simulink model "modelo_final_server"  (R2021a)
settings: Solver=FixedStepAuto  StartTime=0.0  StopTime=inf  FixedStep=0.001  MaxStep=1e-4  RelTol=1e-3
values from neighbouring files (symbols this model uses):
  bah = Meqh*nh*w_posh    (= 720000)    [Data.m]
  bat = Meqt*nt*w_post    (= 675000)    [Data.m]
  bcx = 1000.0    (= 1000)    [Data.m]
  bcy = 500.0    (= 500)    [Data.m]
  beqhd = bh + ((beqh*(rth^2))/(Rd^2))    (= 28800)    [Data.m]
  beqt = bt + (beq_rot*rt^2)/(Rw^2)    (= 27000)    [Data.m]
  bw = 30000.0    (= 30000)    [Data.m]
  cols_centers = [5,10,15,20,25,30,35,40,45]    [Data.m]    (also in generateTrajectory.m = ship.allocate_centers(container.width/2,delta))
  cols_height = [20,26,19,8,26,20,26,23,23]    [Data.m]    (also in generateTrajectory.m = ship.load(container))
  ddxmax = 1    [Data.m]
  ddxmin = -1    [Data.m]
  ddymax = 1    [Data.m]
  ddymin = -1    [Data.m]
  g = 9.80665    [Data.m]    (also in PD_balanceo.m = 9.81)
  Kcy = 1.3e6    (= 1300000)    [Data.m]
  Ksah = Meqh*nh*w_posh^2    (= 4318720.37915)    [Data.m]
  Ksat = Meqt*nt*w_post^2    (= 3088564.26247)    [Data.m]
  Ksiah = Meqh*w_posh^3    (= 10361858.7296)    [Data.m]
  Ksiat = Meqt*w_post^3    (= 5652876.56499)    [Data.m]
  Kw = 1800000.0    (= 1800000)    [Data.m]
  lh0 = yt0 - C_HEIGHT - 5 -(sp_mass * g) / Kw    (= 37.0282779167)    [Data.m]
  max_m = 50000.0    (= 50000)    [Data.m]
  Meqh = Mh + (Jmh*rth^2 + Jd)/Rd^2    (= 48014.2222222)    [Data.m]
  Meqt = mt + (Jw+Jm*rt^2)/(Rw^2)    (= 59008)    [Data.m]
  Rd = 0.75    [Data.m]
  rt = 15.0    (= 15)    [Data.m]    (also in main.m = 0)
  rth = 30.0    (= 30)    [Data.m]
  Rw = 0.5    [Data.m]    (also in main.m = 0)
  sp_mass = 15000.0    (= 15000)    [Data.m]
  w_mt_h = 1000    [Data.m]
  w_mt_i = 1000    [Data.m]
  xmax = 50    [Data.m]
  xt0 = -20    [Data.m]
  yt0 = 45.0    (= 45)    [Data.m]
undefined symbols (not defined in the file or in its folder): yl0
libraries: aerolibanimutils x1, simulink x1
settings Model: Creator=Mariano  LastModifiedBy=facu_
settings SolverCC: ODENIntegrationMethod=ode2

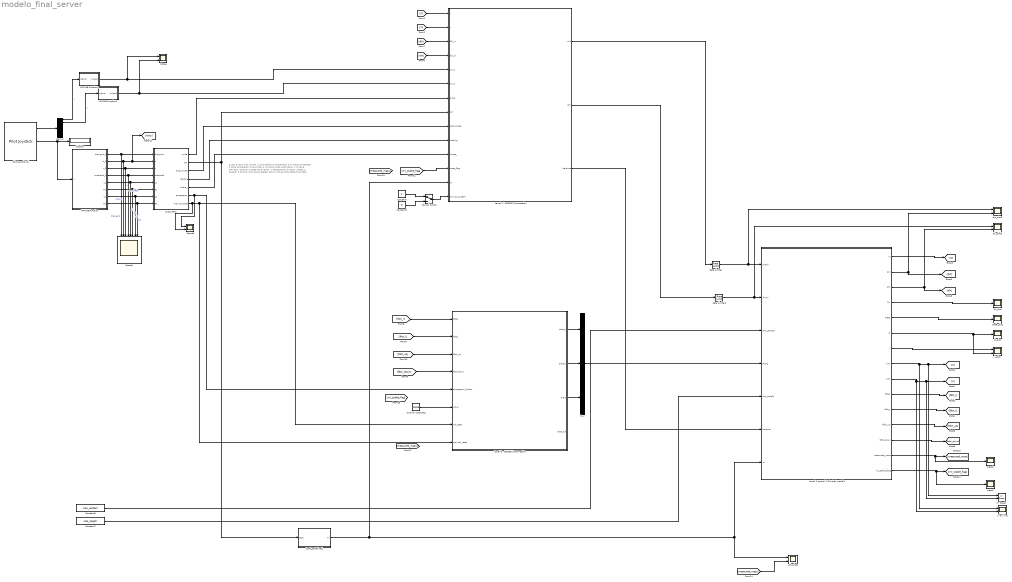
== system modelo_final_server ==
  note: Cycle: Si es 0 ciclo simple, 1 ciclo doble
      | twt (twtistlocks): 0 no tiene contenedor, 1 tiene contenedor.
      | auto_mode: 0 no tiene modo automatico, 1 lo tiene activado.
      | loading: 0 cargando el barco, 1 descargando el barco.
      | where_:1 to_dock, 0 to ship
      | manual_completed: tramo manual ciclo doble finalizado
  Constant : Constant
  Constant1 : Constant  Value=0
  Constant6 : Constant  Value=cols_centers
  Constant7 : Constant  Value=cols_height
  Demux : Demux  Outputs=6
  Display : Display
  Fw_plot : Scope
  Level 0 - CODESYS connection : Subsystem  TreatAsAtomicUnit=on  SystemSampleTime=0.1
  Level 1 - CODESYS connection : Subsystem  TreatAsAtomicUnit=on  SystemSampleTime=0.1
  Level 2 control + Physical model1 : Subsystem
  Load_container1 : Subsystem
  MATLAB Function : MATLAB Function  TreatAsAtomicUnit=on
  MATLAB Function1 : MATLAB Function  TreatAsAtomicUnit=on
  MATLAB Function2 : MATLAB Function  TreatAsAtomicUnit=on
  Manual Switch : ManualSwitch
  Mux : Mux  Inputs=3
  Pilot Joystick All : aerolibanimutils/Pilot Joystick  JoystickID=Joystick1  OutputConfiguration=AllOutputs  SampleTime=1/10
  Rate Limiter : RateLimiter  RisingSlewLimit=ddxmax  FallingSlewLimit=ddxmin  SampleTimeMode=inherited
  Rate Limiter1 : RateLimiter  RisingSlewLimit=ddymax  FallingSlewLimit=ddymin  SampleTimeMode=inherited
  Scope : Scope  NumInputPorts=2
  Scope1 : Scope  NumInputPorts=8
  Scope2 : Scope  NumInputPorts=2
  Subsystem : Subsystem
  XY Graph : simulink/Sinks/XY Graph  xmin=-22  xmax=50  ymin=0  ymax=50  st=-1
  clock for watchdog : DiscretePulseGenerator  PulseType=Time based  Period=1  PulseWidth=50
  dlh_plot1 : Scope  NumInputPorts=2
  dlh_plot2 : Scope  NumInputPorts=2
  dxt_plot3 : Scope  NumInputPorts=2
  l_plot : Scope  NumInputPorts=2
  lh_plot : Scope
  mass1 : Scope
  mass2 : Scope
  theta_plot : Scope
  xl e yl vs t : Scope  NumInputPorts=2
  wires:
  MATLAB Function/8(R2) -> Subsystem/8(R2), Scope1/8  "R2"
  MATLAB Function/7(L2) -> Subsystem/7(L2), Scope1/7  "L2"
  MATLAB Function/2(o_2) -> Scope1/2, [twts], Subsystem/2(o)  "circulo"
  MATLAB Function/3(x_3) -> Scope1/3, Subsystem/3(x)  "x"
  MATLAB Function/4(cuadrado_4) -> Subsystem/4(cuadrado), Scope1/4  "cuadrado"
  Pilot Joystick All/2 -> MATLAB Function/1(u), Display/1
  Pilot Joystick All/1 -> Demux/1
  MATLAB Function/5(L1) -> Subsystem/5(L1), Scope1/5  "L1"
  Demux/1 -> MATLAB Function1/1(signal)  "x"
  Level 1 - CODESYS connection/1(dxt) -> Rate Limiter/1
  Rate Limiter1/1 -> dlh_plot1/1, Level 2 control + Physical model1/2(dlh(t)*)
  Demux/2 -> MATLAB Function2/1(signal)  "y"
  Level 2 control + Physical model1/2(dxt) -> [dxt], dxt_plot3/2
  Constant7/1 -> Level 2 control + Physical model1/5(cols_height)
  Level 1 - CODESYS connection/2(dlh) -> Rate Limiter1/1
  Level 2 control + Physical model1/9(yl(t)) -> xl e yl vs t/2, XY Graph/2, [yl]
  Constant6/1 -> Level 2 control + Physical model1/3(cols_centers)
  Level 2 control + Physical model1/4(Fw) -> Fw_plot/1
  Level 2 control + Physical model1/3(dlh) -> [dlh], dlh_plot1/2
  Level 2 control + Physical model1/6(lh) -> l_plot/2, lh_plot/1
  Level 2 control + Physical model1/7(l) -> l_plot/1
  Level 2 control + Physical model1/1(xt) -> [xt]
  [xl] -> Level 1 - CODESYS connection/2(x)
  Level 2 control + Physical model1/5(theta) -> theta_plot/1
  [yl] -> Level 1 - CODESYS connection/1(y)
  Level 1 - CODESYS connection/3(balance) -> Level 2 control + Physical model1/6(balance)
  MATLAB Function/1(triangulo_1) -> Scope1/1, Subsystem/1(triangulo)  "triangulo"
  MATLAB Function/6(R1) -> Subsystem/6(R1), Scope1/6  "R1"
  Rate Limiter/1 -> dxt_plot3/1, Level 2 control + Physical model1/1(dxt(t)*)
  [dlh] -> Level 1 - CODESYS connection/3(dlh_in)
  Level 2 control + Physical model1/8(xl(t)) -> xl e yl vs t/1, XY Graph/1, [xl]
  [dxt] -> Level 1 - CODESYS connection/4(dxt_in)
  [fdct_r] -> Level 0 - CODESYS connection/1(fdct_r)
  [fdct_l] -> Level 0 - CODESYS connection/2(fdct_l)
  [fdch_down] -> Level 0 - CODESYS connection/4(fdch_down)
  [fdch_up] -> Level 0 - CODESYS connection/3(fdch_up)
  Subsystem/6(emergency) -> Scope2/1, Level 0 - CODESYS connection/5(emergency_button)
  Level 2 control + Physical model1/10(fdct_l) -> [fdct_l]
  Level 2 control + Physical model1/11(fdct_r) -> [fdct_r]
  Level 2 control + Physical model1/12(fdch_up) -> [fdch_up]
  Level 2 control + Physical model1/13(fdch_down) -> [fdch_down]
  Subsystem/7(manual_reset) -> Scope2/2, Level 0 - CODESYS connection/7(wd_reset), Level 0 - CODESYS connection/8(manual_reset)
  Level 0 - CODESYS connection/2(alert_h) -> Mux/2
  Level 0 - CODESYS connection/1(alert_t) -> Mux/1
  Level 0 - CODESYS connection/3(alert) -> Mux/3
  Mux/1 -> Level 2 control + Physical model1/4(alerts)
  Level 2 control + Physical model1/14(measured_mass) -> mass2/1, [measured_mass]
  Level 2 control + Physical model1/15(ml_stable_flag) -> mass1/1, [ml_stable_flag]
  [ml_stable_flag] -> Level 1 - CODESYS connection/12(mass_flag)
  Subsystem/2(twt) -> Load_container1/1(start), Level 1 - CODESYS connection/8(twt)
  Subsystem/1(cycle) -> Level 1 - CODESYS connection/7(cycle)
  Subsystem/3(auto_mode) -> Level 1 - CODESYS connection/9(auto_mode)
  Subsystem/4(loading) -> Level 1 - CODESYS connection/10(loading)
  Subsystem/5(where_) -> Level 1 - CODESYS connection/11(where_)
  Load_container1/1(ml) -> dlh_plot2/1, Level 2 control + Physical model1/7(ml), Level 1 - CODESYS connection/13(ml)
  MATLAB Function2/1(output) -> Scope/2, Level 1 - CODESYS connection/6(joy_h)
  [measured_mass] -> dlh_plot2/2
  clock for watchdog/1 -> Level 0 - CODESYS connection/6(wd_in)
  Manual Switch/1 -> Level 1 - CODESYS connection/14(turn_on_system)
  Constant/1 -> Manual Switch/1
  Constant1/1 -> Manual Switch/2
  MATLAB Function1/1(output) -> Scope/1, Level 1 - CODESYS connection/5(joy_t)

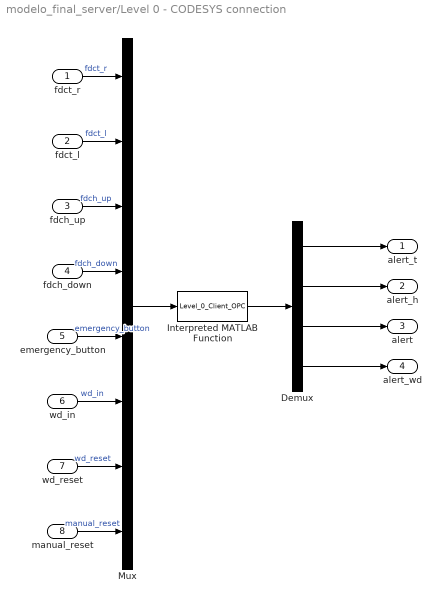
== system modelo_final_server/Level 0 - CODESYS connection ==
  fdct_r : Inport  LockScale=on
  fdct_l : Inport  Port=2  LockScale=on
  fdch_up : Inport  Port=3  LockScale=on
  fdch_down : Inport  Port=4  LockScale=on
  emergency_button : Inport  Port=5  LockScale=on
  wd_in : Inport  Port=6  LockScale=on
  wd_reset : Inport  Port=7  LockScale=on
  manual_reset : Inport  Port=8  LockScale=on
  Demux : Demux
  Interpreted MATLAB Function : MATLABFcn  MATLABFcn=Level_0_Client_OPC  OutputDimensions=4
  Mux : Mux  Inputs=8
  alert_t : Outport  LockScale=on
  alert_h : Outport  Port=2  LockScale=on
  alert : Outport  Port=3  LockScale=on
  alert_wd : Outport  Port=4  LockScale=on
  wires:
  Demux/1 -> alert_t/1
  Demux/2 -> alert_h/1
  Demux/3 -> alert/1
  Demux/4 -> alert_wd/1
  Mux/1 -> Interpreted MATLAB Function/1
  Interpreted MATLAB Function/1 -> Demux/1
  fdct_r/1 -> Mux/1  "fdct_r"
  fdct_l/1 -> Mux/2  "fdct_l"
  fdch_up/1 -> Mux/3  "fdch_up"
  fdch_down/1 -> Mux/4  "fdch_down"
  emergency_button/1 -> Mux/5  "emergency_button"
  wd_in/1 -> Mux/6  "wd_in"
  wd_reset/1 -> Mux/7  "wd_reset"
  manual_reset/1 -> Mux/8  "manual_reset"

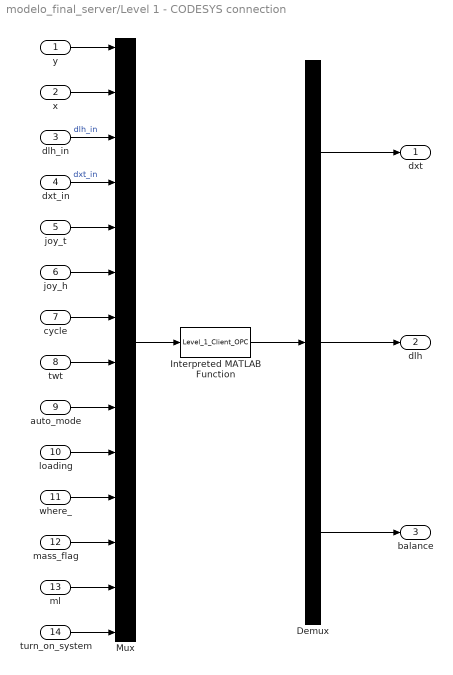
== system modelo_final_server/Level 1 - CODESYS connection ==
  y : Inport
  x : Inport  Port=2
  dlh_in : Inport  Port=3
  dxt_in : Inport  Port=4
  joy_t : Inport  Port=5
  joy_h : Inport  Port=6
  cycle : Inport  Port=7
  twt : Inport  Port=8
  auto_mode : Inport  Port=9
  loading : Inport  Port=10
  where_ : Inport  Port=11
  mass_flag : Inport  Port=12
  ml : Inport  Port=13
  turn_on_system : Inport  Port=14
  Demux : Demux  Outputs=3
  Interpreted MATLAB Function : MATLABFcn  MATLABFcn=Level_1_Client_OPC  OutputDimensions=3
  Mux : Mux  Inputs=14
  dxt : Outport
  dlh : Outport  Port=2
  balance : Outport  Port=3
  wires:
  y/1 -> Mux/1
  x/1 -> Mux/2
  dlh_in/1 -> Mux/3  "dlh_in"
  dxt_in/1 -> Mux/4  "dxt_in"
  joy_t/1 -> Mux/5
  joy_h/1 -> Mux/6
  cycle/1 -> Mux/7
  twt/1 -> Mux/8
  auto_mode/1 -> Mux/9
  loading/1 -> Mux/10
  where_/1 -> Mux/11
  mass_flag/1 -> Mux/12
  ml/1 -> Mux/13
  Mux/1 -> Interpreted MATLAB Function/1
  Interpreted MATLAB Function/1 -> Demux/1
  Demux/1 -> dxt/1
  Demux/3 -> balance/1
  Demux/2 -> dlh/1
  turn_on_system/1 -> Mux/14

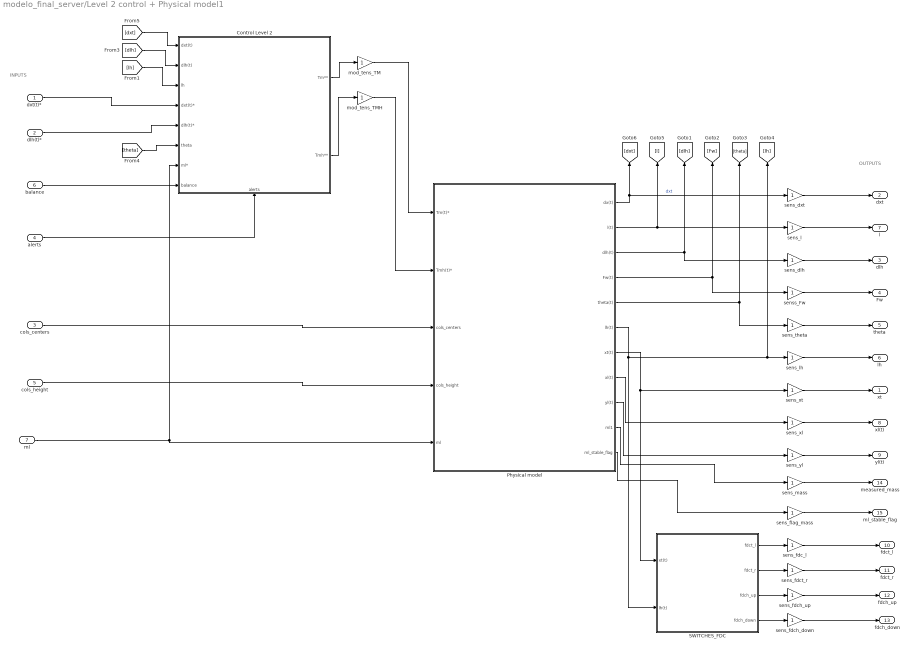
== system modelo_final_server/Level 2 control + Physical model1 ==
  note: OUTPUTS
  note: INPUTS
  dxt(t)* : Inport
  dlh(t)* : Inport  Port=2
  cols_centers : Inport  Port=3
  alerts : Inport  Port=4
  cols_height : Inport  Port=5
  balance : Inport  Port=6
  ml : Inport  Port=7
  Control Level 2 : Subsystem
      settings: PortSchema="{\"entries\":[{\"content\":{\"sides\":[{\"content\":{\"connectorIds\":[\"In1\",\"In2\",\"In3\",\"In4\",\"In5\",\"In6\",\"In7\",\"In8\"]},\"type\":\"ConnectorPlacement.EquallySpacedRectSide\",\"uuid\":\"e38639ea-7b0c-472b-b906-c3080a9fe90e\"},{\"content\":{\"connectorIds\":[\"Out1\",\"Out2\"],\"side\":\"RIGHT\"},\"type\":\"ConnectorPlacement.EquallySpacedRectSide\",\"uuid\":\"f157ca09-fac1-4e54-932c-e4a091123ca7\"},{\"content\":{\"connectorIds\":[],\"side\":\"TOP\"},\"type\":\"ConnectorPlacement.EquallySpacedRectSide\",\"uuid\":\"67ac1266-4733-4780-abf3-e4f9156f2c95\"},{\"content\":{\"connectorIds\":[\"In9\"],\"side\":\"BOTTOM\"},\"type\":\"ConnectorPlacement.EquallySpacedRectSide\",\"uuid\":\"9ec969bf-ffae-45c2-8f7a-57d0a1bfe486\"}]},\"type\":\"ConnectorPlacement.EquallySpacedConnector\",\"uuid\":\"d230347d-5e67-46d6-9931-d869083e937c\"}],\"packageUris\":[\"http://schema.mathworks.com/mf0/Connector/R2020b\"],\"version\":\"1.0\"}"
  Physical model : Subsystem
  SWITCHES_FDC : Subsystem
  mod_tens_TM : Gain
  mod_tens_TMH : Gain
  sens_dlh : Gain
  sens_dxt : Gain
  sens_fdc_l : Gain
  sens_fdch_down : Gain
  sens_fdch_up : Gain
  sens_fdct_r : Gain
  sens_flag_mass : Gain
  sens_l : Gain
  sens_lh : Gain
  sens_mass : Gain
  sens_theta : Gain
  sens_xl : Gain
  sens_xt : Gain
  sens_yl : Gain
  senss_Fw : Gain
  xt : Outport
  dxt : Outport  Port=2
  dlh : Outport  Port=3
  Fw : Outport  Port=4
  theta : Outport  Port=5
  lh : Outport  Port=6
  l : Outport  Port=7
  xl(t) : Outport  Port=8
  yl(t) : Outport  Port=9
  fdct_l : Outport  Port=10
  fdct_r : Outport  Port=11
  fdch_up : Outport  Port=12
  fdch_down : Outport  Port=13
  measured_mass : Outport  Port=14
  ml_stable_flag : Outport  Port=15
  wires:
  Physical model/4(Fw(t)) -> senss_Fw/1, [Fw]
  Physical model/3(dlh(t)) -> sens_dlh/1, [dlh]
  senss_Fw/1 -> Fw/1
  sens_xt/1 -> xt/1
  dlh(t)*/1 -> Control Level 2/5(dlh(t)*)
  Physical model/5(theta(t)) -> sens_theta/1, [theta]
  mod_tens_TMH/1 -> Physical model/2(Tmh(t)*)
  Physical model/1(dx(t)) -> [dxt], sens_dxt/1  "dxt"
  ml/1 -> Control Level 2/7(ml*), Physical model/5(ml)
  Physical model/6(lh(t)) -> sens_lh/1, [lh], SWITCHES_FDC/2(lh(t))
  sens_dlh/1 -> dlh/1
  sens_theta/1 -> theta/1
  Control Level 2/1(Tm**) -> mod_tens_TM/1
  Physical model/2(l(t)) -> [l], sens_l/1
  sens_lh/1 -> lh/1
  sens_dxt/1 -> dxt/1
  Physical model/7(xt(t)) -> sens_xt/1, SWITCHES_FDC/1(xt(t))
  Control Level 2/2(Tmh**) -> mod_tens_TMH/1
  mod_tens_TM/1 -> Physical model/1(Tm(t)*)
  cols_centers/1 -> Physical model/3(cols_centers)
  cols_height/1 -> Physical model/4(cols_height)
  sens_l/1 -> l/1
  [dxt] -> Control Level 2/1(dxt(t))
  [lh] -> Control Level 2/3(lh)
  [dlh] -> Control Level 2/2(dlh(t))
  [theta] -> Control Level 2/6(theta)
  Physical model/9(yl(t)) -> sens_yl/1
  Physical model/8(xl(t)) -> sens_xl/1
  sens_xl/1 -> xl(t)/1
  sens_yl/1 -> yl(t)/1
  balance/1 -> Control Level 2/8(balance)
  SWITCHES_FDC/1(fdct_l) -> sens_fdc_l/1
  SWITCHES_FDC/2(fdct_r) -> sens_fdct_r/1
  SWITCHES_FDC/3(fdch_up) -> sens_fdch_up/1
  SWITCHES_FDC/4(fdch_down) -> sens_fdch_down/1
  sens_fdc_l/1 -> fdct_l/1
  sens_fdct_r/1 -> fdct_r/1
  sens_fdch_up/1 -> fdch_up/1
  sens_fdch_down/1 -> fdch_down/1
  alerts/1 -> Control Level 2/9(alerts)
  dxt(t)*/1 -> Control Level 2/4(dxt(t)*)
  Physical model/10(ml1) -> sens_mass/1
  Physical model/11(ml_stable_flag) -> sens_flag_mass/1
  sens_flag_mass/1 -> ml_stable_flag/1
  sens_mass/1 -> measured_mass/1

== system modelo_final_server/Load_container1 ==
  start : Inport
  Sum : Sum  Inputs=|++
  Switch : Switch  Criteria=u2 > Threshold
  no_container : Constant  Value=0
  random_container_mass : Constant  Value=max_m
  spreader mass : Constant  Value=sp_mass
  ml : Outport
  wires:
  spreader mass/1 -> Sum/2
  Switch/1 -> Sum/1
  Sum/1 -> ml/1
  start/1 -> Switch/2
  random_container_mass/1 -> Switch/1
  no_container/1 -> Switch/3

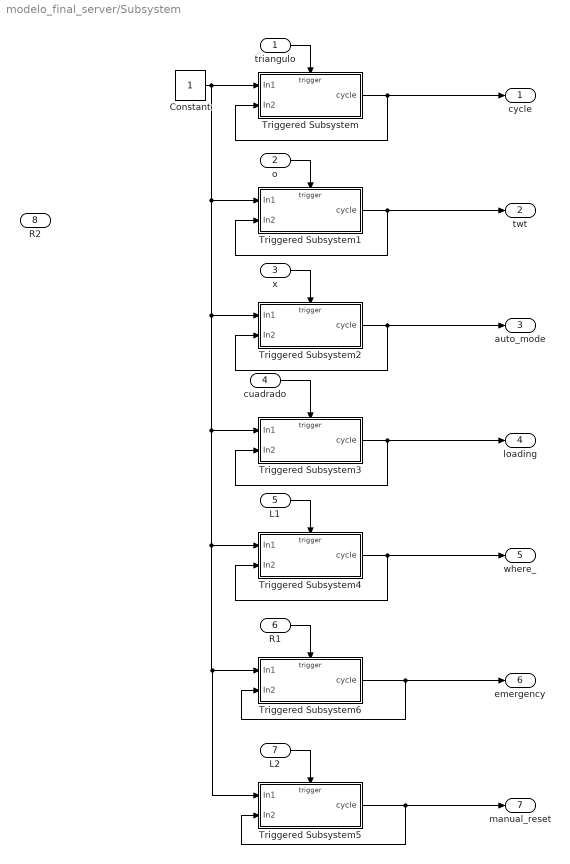
== system modelo_final_server/Subsystem ==
  triangulo : Inport
  o : Inport  Port=2
  x : Inport  Port=3
  cuadrado : Inport  Port=4
  L1 : Inport  Port=5
  R1 : Inport  Port=6
  L2 : Inport  Port=7
  R2 : Inport  Port=8
  Constant : Constant
  Triggered Subsystem : Subsystem  TreatAsAtomicUnit=on
  Triggered Subsystem1 : Subsystem  TreatAsAtomicUnit=on
  Triggered Subsystem2 : Subsystem  TreatAsAtomicUnit=on
  Triggered Subsystem3 : Subsystem  TreatAsAtomicUnit=on
  Triggered Subsystem4 : Subsystem  TreatAsAtomicUnit=on
  Triggered Subsystem5 : Subsystem  TreatAsAtomicUnit=on
  Triggered Subsystem6 : Subsystem  TreatAsAtomicUnit=on
  cycle : Outport
  twt : Outport  Port=2
  auto_mode : Outport  Port=3
  loading : Outport  Port=4
  where_ : Outport  Port=5
  emergency : Outport  Port=6
  manual_reset : Outport  Port=7
  wires:
  triangulo/1 -> Triggered Subsystem/Trigger
  Triggered Subsystem/1(cycle) -> Triggered Subsystem/2(In2), cycle/1
  Triggered Subsystem1/1(cycle) -> twt/1, Triggered Subsystem1/2(In2)
  o/1 -> Triggered Subsystem1/Trigger
  Triggered Subsystem2/1(cycle) -> auto_mode/1, Triggered Subsystem2/2(In2)
  x/1 -> Triggered Subsystem2/Trigger
  Triggered Subsystem3/1(cycle) -> loading/1, Triggered Subsystem3/2(In2)
  cuadrado/1 -> Triggered Subsystem3/Trigger
  Triggered Subsystem4/1(cycle) -> where_/1, Triggered Subsystem4/2(In2)
  L1/1 -> Triggered Subsystem4/Trigger
  R1/1 -> Triggered Subsystem6/Trigger
  Triggered Subsystem6/1(cycle) -> Triggered Subsystem6/2(In2), emergency/1
  Triggered Subsystem5/1(cycle) -> Triggered Subsystem5/2(In2), manual_reset/1
  L2/1 -> Triggered Subsystem5/Trigger
  Constant/1 -> Triggered Subsystem3/1(In1), Triggered Subsystem5/1(In1), Triggered Subsystem6/1(In1), Triggered Subsystem4/1(In1), Triggered Subsystem2/1(In1), Triggered Subsystem1/1(In1), Triggered Subsystem/1(In1)

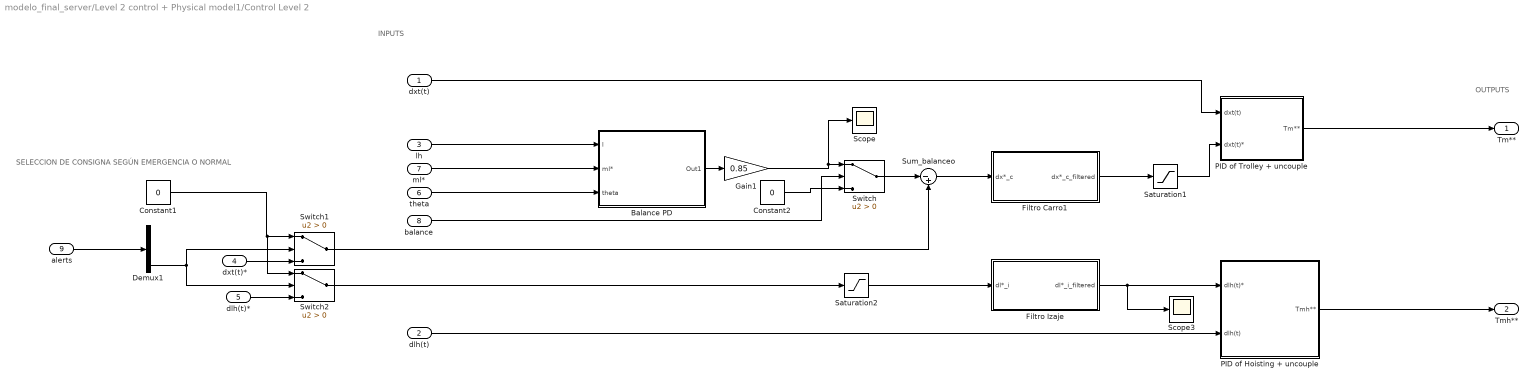
== system modelo_final_server/Level 2 control + Physical model1/Control Level 2 ==
  note: SELECCION DE CONSIGNA SEGÚN EMERGENCIA O NORMAL
  note: OUTPUTS
  note: INPUTS
  dxt(t) : Inport
  dlh(t) : Inport  Port=2
  lh : Inport  Port=3
  dxt(t)* : Inport  Port=4
  dlh(t)* : Inport  Port=5
  theta : Inport  Port=6
  ml* : Inport  Port=7
  balance : Inport  Port=8
  alerts : Inport  Port=9
  Balance PD : Subsystem
  Constant1 : Constant  Value=0
  Constant2 : Constant  Value=0
  Demux1 : Demux  Outputs=3
  Filtro Carro1 : Subsystem
  Filtro Izaje : Subsystem
  Gain1 : Gain  Gain=0.85
  "PID of Hoisting + uncouple " : Subsystem
  "PID of Trolley + uncouple " : Subsystem
  Saturation1 : Saturate  UpperLimit=4  LowerLimit=-4
  Saturation2 : Saturate  UpperLimit=3  LowerLimit=-3
  Scope : Scope
  Scope3 : Scope
  Sum_balanceo : Sum  Inputs=|-+
  Switch : Switch  Criteria=u2 > Threshold
  Switch1 : Switch  Criteria=u2 > Threshold
  Switch2 : Switch  Criteria=u2 > Threshold
  Tm** : Outport
  Tmh** : Outport  Port=2
  wires:
  "PID of Trolley + uncouple "/1(Tm**) -> Tm**/1
  dxt(t)/1 -> "PID of Trolley + uncouple "/1(dxt(t))
  "PID of Hoisting + uncouple "/1(Tmh**) -> Tmh**/1
  theta/1 -> Balance PD/3(theta)
  dlh(t)/1 -> "PID of Hoisting + uncouple "/2(dlh(t))
  Filtro Izaje/1(dl*_i_filtered) -> Scope3/1, "PID of Hoisting + uncouple "/1(dlh(t)*)
  balance/1 -> Switch/2
  Constant2/1 -> Switch/3
  ml*/1 -> Balance PD/2(ml*)
  lh/1 -> Balance PD/1(l)
  Switch/1 -> Sum_balanceo/1
  Balance PD/1(Out1) -> Gain1/1
  Sum_balanceo/1 -> Filtro Carro1/1(dx*_c)
  Saturation2/1 -> Filtro Izaje/1(dl*_i)
  Switch1/1 -> Sum_balanceo/2
  Gain1/1 -> Switch/1, Scope/1
  Saturation1/1 -> "PID of Trolley + uncouple "/2(dxt(t)*)
  Filtro Carro1/1(dx*_c_filtered) -> Saturation1/1
  alerts/1 -> Demux1/1
  dxt(t)*/1 -> Switch1/3
  Constant1/1 -> Switch2/1, Switch1/1
  Switch2/1 -> Saturation2/1
  dlh(t)*/1 -> Switch2/3
  Demux1/3 -> Switch1/2, Switch2/2

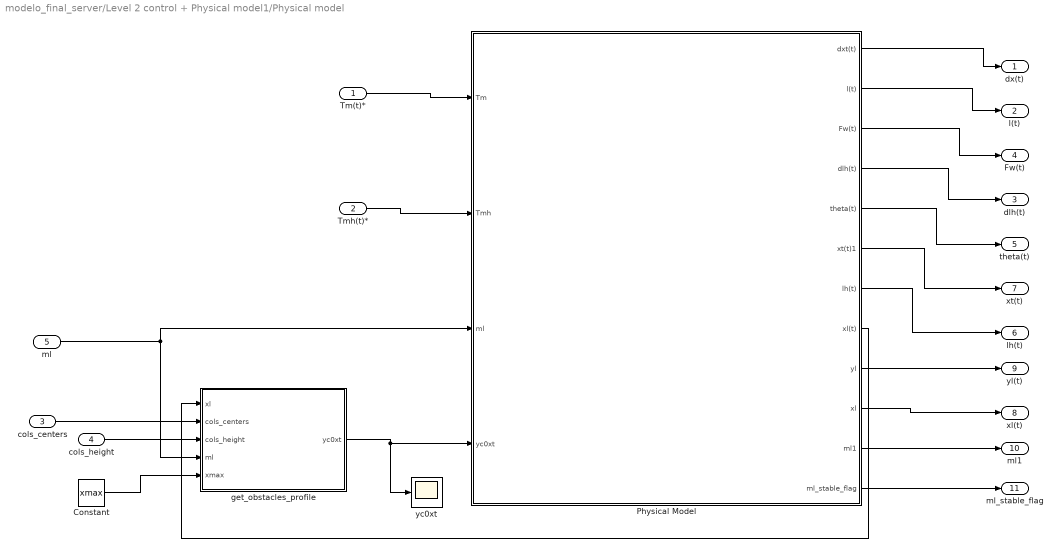
== system modelo_final_server/Level 2 control + Physical model1/Physical model ==
  Tm(t)* : Inport
  Tmh(t)* : Inport  Port=2
  cols_centers : Inport  Port=3
  cols_height : Inport  Port=4
  ml : Inport  Port=5
  Constant : Constant  Value=xmax
  Physical Model : Subsystem
  get_obstacles_profile : MATLAB Function  TreatAsAtomicUnit=on
  yc0xt : Scope
  dx(t) : Outport
  l(t) : Outport  Port=2
  dlh(t) : Outport  Port=3
  Fw(t) : Outport  Port=4
  theta(t) : Outport  Port=5
  lh(t) : Outport  Port=6
  xt(t) : Outport  Port=7
  xl(t) : Outport  Port=8
  yl(t) : Outport  Port=9
  ml1 : Outport  Port=10
  ml_stable_flag : Outport  Port=11
  wires:
  Physical Model/4(dlh(t)) -> dlh(t)/1
  Physical Model/2(l(t)) -> l(t)/1
  Physical Model/1(dxt(t)) -> dx(t)/1
  Physical Model/3(Fw(t)) -> Fw(t)/1
  Physical Model/5(theta(t)) -> theta(t)/1
  Physical Model/6(xt(t)1) -> xt(t)/1
  Physical Model/7(lh(t)) -> lh(t)/1
  Tmh(t)*/1 -> Physical Model/2(Tmh)
  Tm(t)*/1 -> Physical Model/1(Tm)
  ml/1 -> get_obstacles_profile/4(ml), Physical Model/3(ml)
  get_obstacles_profile/1(yc0xt) -> yc0xt/1, Physical Model/4(yc0xt)
  Physical Model/8(xl(t)) -> get_obstacles_profile/1(xl)
  cols_centers/1 -> get_obstacles_profile/2(cols_centers)
  cols_height/1 -> get_obstacles_profile/3(cols_height)
  Physical Model/10(xl) -> xl(t)/1
  Physical Model/9(yl) -> yl(t)/1
  Constant/1 -> get_obstacles_profile/5(xmax)
  Physical Model/11(ml1) -> ml1/1
  Physical Model/12(ml_stable_flag) -> ml_stable_flag/1

== system modelo_final_server/Level 2 control + Physical model1/SWITCHES_FDC ==
  xt(t) : Inport
  lh(t) : Inport  Port=2
  MATLAB Function : MATLAB Function  TreatAsAtomicUnit=on
  MATLAB Function1 : MATLAB Function  TreatAsAtomicUnit=on
  fdct_l : Outport
  fdct_r : Outport  Port=2
  fdch_up : Outport  Port=3
  fdch_down : Outport  Port=4
  wires:
  xt(t)/1 -> MATLAB Function/1(xt)
  MATLAB Function/1(fdct_l) -> fdct_l/1
  MATLAB Function/2(fdct_r) -> fdct_r/1
  lh(t)/1 -> MATLAB Function1/1(lh)
  MATLAB Function1/1(fdch_up) -> fdch_up/1
  MATLAB Function1/2(fdch_down) -> fdch_down/1

== system modelo_final_server/Subsystem/Triggered Subsystem ==
  In1 : Inport
  In2 : Inport  Port=2  LatchByDelayingOutsideSignal=on
  Trigger : TriggerPort  VariantControl=(inherit)
  Sum : Sum  Inputs=|+-
  cycle : Outport
  wires:
  In1/1 -> Sum/1
  In2/1 -> Sum/2
  Sum/1 -> cycle/1

== system modelo_final_server/Subsystem/Triggered Subsystem1 ==
  In1 : Inport
  In2 : Inport  Port=2  LatchByDelayingOutsideSignal=on
  Trigger : TriggerPort  VariantControl=(inherit)
  Sum : Sum  Inputs=|+-
  cycle : Outport
  wires:
  In1/1 -> Sum/1
  In2/1 -> Sum/2
  Sum/1 -> cycle/1

== system modelo_final_server/Subsystem/Triggered Subsystem2 ==
  In1 : Inport
  In2 : Inport  Port=2  LatchByDelayingOutsideSignal=on
  Trigger : TriggerPort  VariantControl=(inherit)
  Sum : Sum  Inputs=|+-
  cycle : Outport
  wires:
  In1/1 -> Sum/1
  In2/1 -> Sum/2
  Sum/1 -> cycle/1

== system modelo_final_server/Subsystem/Triggered Subsystem3 ==
  In1 : Inport
  In2 : Inport  Port=2  LatchByDelayingOutsideSignal=on
  Trigger : TriggerPort  VariantControl=(inherit)
  Sum : Sum  Inputs=|+-
  cycle : Outport
  wires:
  In1/1 -> Sum/1
  In2/1 -> Sum/2
  Sum/1 -> cycle/1

== system modelo_final_server/Subsystem/Triggered Subsystem4 ==
  In1 : Inport
  In2 : Inport  Port=2  LatchByDelayingOutsideSignal=on
  Trigger : TriggerPort  VariantControl=(inherit)
  Sum : Sum  Inputs=|+-
  cycle : Outport
  wires:
  In1/1 -> Sum/1
  In2/1 -> Sum/2
  Sum/1 -> cycle/1

== system modelo_final_server/Subsystem/Triggered Subsystem5 ==
  In1 : Inport
  In2 : Inport  Port=2  LatchByDelayingOutsideSignal=on
  Trigger : TriggerPort  VariantControl=(inherit)
  Sum : Sum  Inputs=|+-
  cycle : Outport
  wires:
  In1/1 -> Sum/1
  In2/1 -> Sum/2
  Sum/1 -> cycle/1

== system modelo_final_server/Subsystem/Triggered Subsystem6 ==
  In1 : Inport
  In2 : Inport  Port=2  LatchByDelayingOutsideSignal=on
  Trigger : TriggerPort  VariantControl=(inherit)
  Sum : Sum  Inputs=|+-
  cycle : Outport
  wires:
  In1/1 -> Sum/1
  In2/1 -> Sum/2
  Sum/1 -> cycle/1

== system modelo_final_server/Level 2 control + Physical model1/Control Level 2/Balance PD ==
  l : Inport
  ml* : Inport  Port=2
  theta : Inport  Port=3
  Constant : Constant  Value=Meqt
  Derivative : Derivative
  Ganancias Control : MATLAB Function  TreatAsAtomicUnit=on
  Product : Product
  Product1 : Product
  Sum : Sum  Inputs=|-+
  Sum1 : Sum  Inputs=|++
  Wn : Subsystem
  theta_consigna : Constant  Value=0
  Out1 : Outport
  wires:
  l/1 -> Ganancias Control/4(lh), Wn/1(In2)
  ml*/1 -> Wn/2(In3), Ganancias Control/2(ml)
  Sum1/1 -> Out1/1
  theta_consigna/1 -> Sum/2
  theta/1 -> Sum/1
  Constant/1 -> Ganancias Control/1(Mt)
  Ganancias Control/1(Kp) -> Product/1
  Sum/1 -> Product/2, Derivative/1
  Ganancias Control/2(Kd) -> Product1/1
  Wn/1(Wn) -> Ganancias Control/3(Wn)
  Derivative/1 -> Product1/2
  Product1/1 -> Sum1/2
  Product/1 -> Sum1/1

== system modelo_final_server/Level 2 control + Physical model1/Control Level 2/Filtro Carro1 ==
  dx*_c : Inport
  2 : Gain  Gain=10
  Rate Limiter1 : RateLimiter  RisingSlewLimit=ddxmax  FallingSlewLimit=ddxmin  SampleTimeMode=inherited
  Sum3 : Sum  Inputs=|+-
  dl_h(t)2 : Integrator
  dx*_c_filtered : Outport  VectorParamsAs1DForOutWhenUnconnected=off
  wires:
  Sum3/1 -> dl_h(t)2/1
  2/1 -> dx*_c_filtered/1, Sum3/2
  dx*_c/1 -> Rate Limiter1/1
  dl_h(t)2/1 -> 2/1
  Rate Limiter1/1 -> Sum3/1

== system modelo_final_server/Level 2 control + Physical model1/Control Level 2/Filtro Izaje ==
  dl*_i : Inport
  1 : Gain  Gain=10
  Rate Limiter1 : RateLimiter  RisingSlewLimit=ddymax  FallingSlewLimit=ddymin  SampleTimeMode=inherited
  Sum4 : Sum  Inputs=|+-
  dl_h(t)1 : Integrator
  dl*_i_filtered : Outport  VectorParamsAs1DForOutWhenUnconnected=off
  wires:
  dl_h(t)1/1 -> 1/1
  1/1 -> dl*_i_filtered/1, Sum4/2
  Sum4/1 -> dl_h(t)1/1
  dl*_i/1 -> Rate Limiter1/1
  Rate Limiter1/1 -> Sum4/1

== system modelo_final_server/Level 2 control + Physical model1/Control Level 2/PID of Hoisting + uncouple  ==
  dlh(t)* : Inport
  dlh(t) : Inport  Port=2
  Integrator : Integrator
  Integrator1 : Integrator
  Ksah : Gain  Gain=Ksah
  Ksiah : Gain  Gain=Ksiah
  Rd/rth : Gain  Gain=Rd/rth
  Sum : Sum  Inputs=|+-
  Sum1 : Sum  Inputs=+++
  Sum2 : Sum  Inputs=|++
  Transfer Fcn : TransferFcn  Numerator=[w_mt_h]  Denominator=[1 w_mt_h]
  bah : Gain  Gain=bah
  beqhd : Gain  Gain=beqhd
  Tmh** : Outport
  wires:
  Sum/1 -> bah/1, Integrator/1  "errot_dxh(t)"
  dlh(t)*/1 -> Sum/1
  Sum1/1 -> Sum2/1
  dlh(t)/1 -> Sum/2, beqhd/1
  Integrator/1 -> Integrator1/1, Ksah/1
  bah/1 -> Sum1/3
  Ksah/1 -> Sum1/2
  Integrator1/1 -> Ksiah/1
  Ksiah/1 -> Sum1/1
  beqhd/1 -> Rd/rth/1
  Sum2/1 -> Transfer Fcn/1
  Rd/rth/1 -> Sum2/2
  Transfer Fcn/1 -> Tmh**/1

== system modelo_final_server/Level 2 control + Physical model1/Control Level 2/PID of Trolley + uncouple  ==
  dxt(t) : Inport
  dxt(t)* : Inport  Port=2
  Integrator : Integrator
  Integrator1 : Integrator
  Ksat : Gain  Gain=Ksat
  Ksiat : Gain  Gain=Ksiat
  Rw/rt : Gain  Gain=Rw/rt
  Sum : Sum  Inputs=|+-
  Sum1 : Sum  Inputs=+++
  Sum2 : Sum  Inputs=|++
  Transfer Fcn : TransferFcn  Numerator=[w_mt_i]  Denominator=[1 w_mt_i]
  bat : Gain  Gain=bat
  beqt : Gain  Gain=beqt
  Tm** : Outport
  wires:
  Sum/1 -> bat/1, Integrator/1  "error_dxt(t)"
  dxt(t)*/1 -> Sum/1
  dxt(t)/1 -> Sum/2, beqt/1
  Integrator/1 -> Integrator1/1, Ksat/1
  bat/1 -> Sum1/3
  Ksat/1 -> Sum1/2
  Integrator1/1 -> Ksiat/1
  Ksiat/1 -> Sum1/1
  beqt/1 -> Rw/rt/1
  Sum1/1 -> Sum2/1
  Rw/rt/1 -> Sum2/2
  Sum2/1 -> Transfer Fcn/1
  Transfer Fcn/1 -> Tm**/1

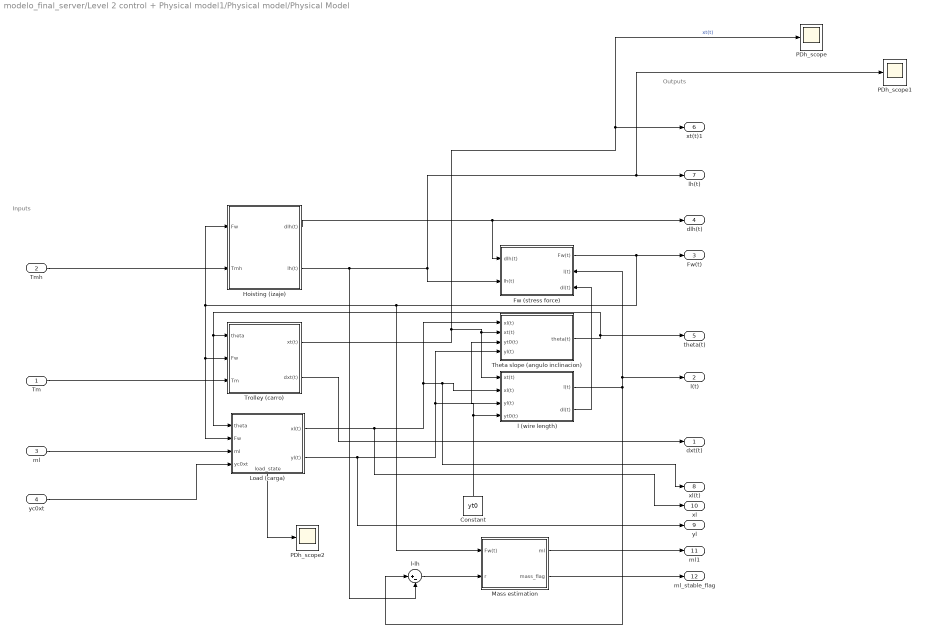
== system modelo_final_server/Level 2 control + Physical model1/Physical model/Physical Model ==
  note: Inputs
  note: Outputs
  Tm : Inport
  Tmh : Inport  Port=2
  ml : Inport  Port=3
  yc0xt : Inport  Port=4
  Constant : Constant  Value=yt0
  Fw (stress force) : Subsystem
      settings: PortSchema="{\"entries\":[{\"content\":{\"sides\":[{\"content\":{\"connectorIds\":[\"In1\",\"In2\"]},\"type\":\"ConnectorPlacement.EquallySpacedRectSide\",\"uuid\":\"ba23d8a5-df88-4a98-9228-1a95ef0572d6\"},{\"content\":{\"connectorIds\":[\"Out1\",\"In3\",\"In4\"],\"side\":\"RIGHT\"},\"type\":\"ConnectorPlacement.EquallySpacedRectSide\",\"uuid\":\"c1b2cc2a-1d19-40da-89ec-405abbf25b58\"},{\"content\":{\"connectorIds\":[],\"side\":\"TOP\"},\"type\":\"ConnectorPlacement.EquallySpacedRectSide\",\"uuid\":\"8c283652-7118-429a-8320-3bc0966db205\"}]},\"type\":\"ConnectorPlacement.EquallySpacedConnector\",\"uuid\":\"7ebc4a5f-6f80-4333-9ee6-9a21b2f2a5d0\"}],\"packageUris\":[\"http://schema.mathworks.com/mf0/Connector/R2020b\"],\"version\":\"1.0\"}"
  Hoisting (izaje) : Subsystem
  Load (carga) : Subsystem
      settings: PortSchema="{\"entries\":[{\"content\":{\"sides\":[{\"content\":{\"connectorIds\":[\"In1\",\"In2\",\"In3\",\"In4\"]},\"type\":\"ConnectorPlacement.EquallySpacedRectSide\",\"uuid\":\"37592506-3a6b-4567-92e8-42290e8eeea3\"},{\"content\":{\"connectorIds\":[\"Out1\",\"Out2\"],\"side\":\"RIGHT\"},\"type\":\"ConnectorPlacement.EquallySpacedRectSide\",\"uuid\":\"0ecb02fc-3423-4f4d-ad91-2cd2f59fe210\"},{\"content\":{\"connectorIds\":[],\"side\":\"TOP\"},\"type\":\"ConnectorPlacement.EquallySpacedRectSide\",\"uuid\":\"e98f0cef-87c8-4aed-91c0-03b7690ae30e\"},{\"content\":{\"connectorIds\":[\"Out3\"],\"side\":\"BOTTOM\"},\"type\":\"ConnectorPlacement.EquallySpacedRectSide\",\"uuid\":\"e16fbcf8-4df1-4bb9-aaa8-254f3178aeca\"}]},\"type\":\"ConnectorPlacement.EquallySpacedConnector\",\"uuid\":\"38642e74-d943-4236-849b-c2d295c3b31e\"}],\"packageUris\":[\"http://schema.mathworks.com/mf0/Connector/R2020b\"],\"version\":\"1.0\"}"
  Mass estimation : Subsystem
  PDh_scope : Scope
  PDh_scope1 : Scope
  PDh_scope2 : Scope
  Theta slope (angulo inclinacion) : Subsystem
  Trolley (carro) : Subsystem
  l (wire length) : Subsystem
  l-lh : Sum  Inputs=|+-
  dxt(t) : Outport
  l(t) : Outport  Port=2
  Fw(t) : Outport  Port=3
  dlh(t) : Outport  Port=4
  theta(t) : Outport  Port=5
  xt(t)1 : Outport  Port=6
  lh(t) : Outport  Port=7
  xl(t) : Outport  Port=8
  yl : Outport  Port=9
  xl : Outport  Port=10
  ml1 : Outport  Port=11
  ml_stable_flag : Outport  Port=12
  wires:
  Theta slope (angulo inclinacion)/1(theta(t)) -> theta(t)/1, Load (carga)/1(theta), Trolley (carro)/1(theta)
  Load (carga)/1(xl(t)) -> xl/1, xl(t)/1, l (wire length)/2(xl(t)), Theta slope (angulo inclinacion)/1(xl(t))
  Trolley (carro)/1(xt(t)) -> PDh_scope/1, xt(t)1/1, l (wire length)/1(xt(t)), Theta slope (angulo inclinacion)/2(xt(t))  "xt(t)"
  Constant/1 -> Theta slope (angulo inclinacion)/3(yt0(t)), l (wire length)/4(yt0(t))
  Load (carga)/2(yl(t)) -> yl/1, Theta slope (angulo inclinacion)/4(yl(t)), l (wire length)/3(yl(t))
  ml/1 -> Load (carga)/3(ml)
  l (wire length)/2(dl(t)) -> Fw (stress force)/4(dl(t))
  Tmh/1 -> Hoisting (izaje)/2(Tmh)
  Tm/1 -> Trolley (carro)/3(Tm)
  Hoisting (izaje)/1(dlh(t)) -> Fw (stress force)/1(dlh(t)), dlh(t)/1
  Trolley (carro)/2(dxt(t)) -> dxt(t)/1
  yc0xt/1 -> Load (carga)/4(yc0xt)
  Load (carga)/3(load_state) -> PDh_scope2/1
  Mass estimation/1(ml) -> ml1/1
  Mass estimation/2(mass_flag) -> ml_stable_flag/1
  Fw (stress force)/1(Fw(t)) -> Fw(t)/1, Mass estimation/1(Fw(t)), Load (carga)/2(Fw), Trolley (carro)/2(Fw), Hoisting (izaje)/1(Fw)
  l-lh/1 -> Mass estimation/2(r)
  Hoisting (izaje)/2(lh(t)) -> l-lh/2, Fw (stress force)/2(lh(t)), PDh_scope1/1, lh(t)/1
  l (wire length)/1(l(t)) -> l(t)/1, Fw (stress force)/3(l(t)), l-lh/1

== system modelo_final_server/Level 2 control + Physical model1/Control Level 2/Balance PD/Wn ==
  In2 : Inport
  In3 : Inport  Port=2
  Constant : Constant  Value=Meqt
  Constant1 : Constant  Value=Meqt*9.81
  Divide : Product  Inputs=*/
  Product : Product
  Sqrt : Sqrt  SaturateOnIntegerOverflow=on
  Sum : Sum  Inputs=|++
  Wn : Outport
  wires:
  Product/1 -> Divide/2
  Constant1/1 -> Divide/1
  Divide/1 -> Sqrt/1
  Sqrt/1 -> Wn/1
  Sum/1 -> Product/1
  In2/1 -> Product/2
  In3/1 -> Sum/2
  Constant/1 -> Sum/1

== system modelo_final_server/Level 2 control + Physical model1/Physical model/Physical Model/Fw (stress force) ==
  note: Carga suspendida
  note: Carga apoyada
  dlh(t) : Inport
  lh(t) : Inport  Port=2
  l(t) : Inport  Port=3
  dl(t) : Inport  Port=4
  Kw : Gain  Gain=Kw
  Kw2 : Gain  Gain=bw
  Sum1 : Sum  Inputs=|+-
  Sum2 : Sum  Inputs=|++
  Sum3 : Sum  Inputs=|+-
  Sum5 : Sum  Inputs=|+-
  Switch : Switch  Criteria=u2 > Threshold
  bw1 : Gain  Gain=bw
  Fw(t) : Outport
  wires:
  l(t)/1 -> Sum1/1
  lh(t)/1 -> Sum1/2
  Sum1/1 -> Switch/2, Kw/1
  Sum3/1 -> bw1/1
  bw1/1 -> Sum2/2
  Kw/1 -> Sum2/1
  Sum2/1 -> Switch/1
  Sum5/1 -> Kw2/1
  dlh(t)/1 -> Sum5/2, Sum3/2
  dl(t)/1 -> Sum5/1, Sum3/1
  Kw2/1 -> Switch/3
  Switch/1 -> Fw(t)/1

== system modelo_final_server/Level 2 control + Physical model1/Physical model/Physical Model/Hoisting (izaje) ==
  Fw : Inport
  Tmh : Inport  Port=2
  "   2" : Constant  Value=45-cols_height(9)
  Constant : Constant  Value=lh0
  Integrator : Integrator
  Integrator1 : Integrator  InitialConditionSource=external
  Manual Switch : ManualSwitch
  Meqh : Gain  Gain=1/Meqh
  Sum : Sum  Inputs=++-
  beqh : Gain  Gain=beqhd
  rth/Rd : Gain  Gain=rth/Rd
  dlh(t) : Outport
  lh(t) : Outport  Port=2
  wires:
  Fw/1 -> Sum/1
  Tmh/1 -> rth/Rd/1
  rth/Rd/1 -> Sum/2
  Sum/1 -> Meqh/1  "ddlh(t)"
  Meqh/1 -> Integrator/1
  Integrator/1 -> dlh(t)/1, beqh/1, Integrator1/1  "dlh(t)"
  Integrator1/1 -> lh(t)/1  "lh(t)"
  beqh/1 -> Sum/3
  "   2"/1 -> Manual Switch/2
  Constant/1 -> Manual Switch/1
  Manual Switch/1 -> Integrator1/2

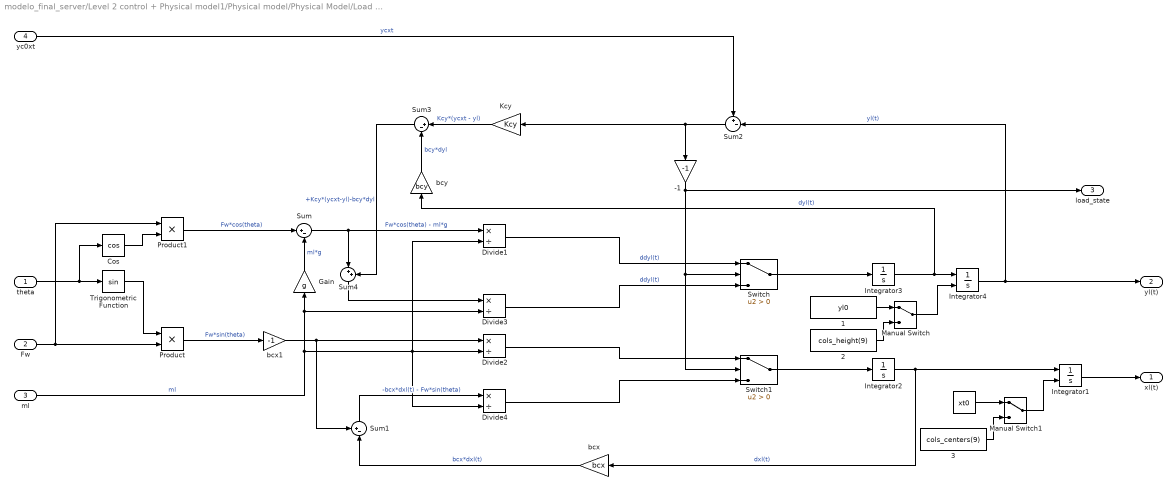
== system modelo_final_server/Level 2 control + Physical model1/Physical model/Physical Model/Load (carga) ==
  theta : Inport
  Fw : Inport  Port=2
  ml : Inport  Port=3
  yc0xt : Inport  Port=4
  "   " : Constant  Value=xt0
  "   1" : Constant  Value=yl0
  "   2" : Constant  Value=cols_height(9)
  "   3" : Constant  Value=cols_centers(9)
  -1 : Gain  Gain=-1
  Cos : Trigonometry  Operator=cos
  Divide{1..4} (4 alike) : Product  Inputs=*/
  Gain : Gain  Gain=g
  Integrator1 : Integrator  InitialConditionSource=external
  Integrator2 : Integrator
  Integrator3 : Integrator
  Integrator4 : Integrator  InitialConditionSource=external
  Kcy : Gain  Gain=Kcy
  Manual Switch : ManualSwitch
  Manual Switch1 : ManualSwitch
  Product : Product
  Product1 : Product
  Sum : Sum  Inputs=|+-
  Sum1 : Sum  Inputs=+-|
  Sum2 : Sum  Inputs=+-|
  Sum3 : Sum  Inputs=|+-
  Sum4 : Sum  Inputs=|++
  Switch : Switch  Criteria=u2 > Threshold
  Switch1 : Switch  Criteria=u2 > Threshold
  Trigonometric Function : Trigonometry
  bcx : Gain  Gain=bcx
  bcx1 : Gain  Gain=-1
  bcy : Gain  Gain=bcy
  xl(t) : Outport
  yl(t) : Outport  Port=2
  load_state : Outport  Port=3
  wires:
  theta/1 -> Trigonometric Function/1, Cos/1
  Trigonometric Function/1 -> Product/1
  Fw/1 -> Product/2, Product1/1
  Integrator1/1 -> xl(t)/1
  Integrator2/1 -> bcx/1, Integrator1/1  "dxl(t)"
  ml/1 -> Divide4/2, Divide2/2, Divide1/2, Divide3/2, Gain/1  "ml"
  Product/1 -> bcx1/1  "Fw*sin(theta)"
  Cos/1 -> Product1/2
  Product1/1 -> Sum/1  "Fw*cos(theta)"
  Sum/1 -> Sum4/1, Divide1/1  "Fw*cos(theta) - ml*g"
  Integrator3/1 -> bcy/1, Integrator4/1  "dyl(t)"
  Integrator4/1 -> Sum2/2, yl(t)/1  "yl(t)"
  Gain/1 -> Sum/2  "ml*g"
  Divide1/1 -> Switch/1  "ddyl(t)"
  Switch/1 -> Integrator3/1
  Switch1/1 -> Integrator2/1
  Divide2/1 -> Switch1/1
  Divide4/1 -> Switch1/3
  Divide3/1 -> Switch/3  "ddyl(t)"
  bcx1/1 -> Sum1/1, Divide2/1
  bcx/1 -> Sum1/2  "bcx*dxl(t)"
  Sum1/1 -> Divide4/1  "-bcx*dxl(t) - Fw*sin(theta)"
  Sum2/1 -> Kcy/1, -1/1
  yc0xt/1 -> Sum2/1  "ycxt"
  Kcy/1 -> Sum3/1  "Kcy*(ycxt - yl)"
  bcy/1 -> Sum3/2  "bcy*dyl"
  Sum4/1 -> Divide3/1
  Sum3/1 -> Sum4/2  "+Kcy*(ycxt-yl)-bcy*dyl"
  -1/1 -> load_state/1, Switch1/2, Switch/2
  "   1"/1 -> Manual Switch/1
  Manual Switch/1 -> Integrator4/2
  "   "/1 -> Manual Switch1/1
  Manual Switch1/1 -> Integrator1/2
  "   2"/1 -> Manual Switch/2
  "   3"/1 -> Manual Switch1/2

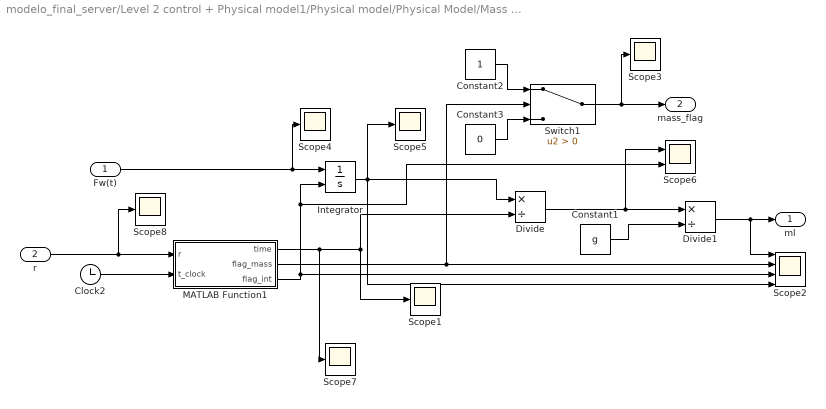
== system modelo_final_server/Level 2 control + Physical model1/Physical model/Physical Model/Mass estimation ==
  Fw(t) : Inport
  r : Inport  Port=2
  Clock2 : Clock
  Constant1 : Constant  Value=g
  Constant2 : Constant
  Constant3 : Constant  Value=0
  Divide : Product  Inputs=*/
  Divide1 : Product  Inputs=*/
  Integrator : Integrator  ExternalReset=rising
  MATLAB Function1 : MATLAB Function  TreatAsAtomicUnit=on
  Scope{1,3..5,7..8} (6 alike) : Scope
  Scope2 : Scope  NumInputPorts=4
  Scope6 : Scope  NumInputPorts=2
  Switch1 : Switch  Criteria=u2 > Threshold
  ml : Outport
  mass_flag : Outport  Port=2
  wires:
  Constant1/1 -> Divide1/2
  Divide1/1 -> Scope2/1, ml/1
  Switch1/1 -> Scope3/1, mass_flag/1
  Constant2/1 -> Switch1/1
  Constant3/1 -> Switch1/3
  Fw(t)/1 -> Integrator/1, Scope4/1
  r/1 -> Scope8/1, MATLAB Function1/1(r)
  Integrator/1 -> Divide/1, Scope2/4, Scope5/1
  Divide/1 -> Scope6/1, Divide1/1
  MATLAB Function1/1(time) -> Scope7/1, Scope1/1, Divide/2
  Clock2/1 -> MATLAB Function1/2(t_clock)
  MATLAB Function1/2(flag_mass) -> Switch1/2, Scope2/2
  MATLAB Function1/3(flag_int) -> Scope2/3, Scope6/2, Integrator/2

== system modelo_final_server/Level 2 control + Physical model1/Physical model/Physical Model/Theta slope (angulo inclinacion) ==
  xl(t) : Inport
  xt(t) : Inport  Port=2
  yt0(t) : Inport  Port=3
  yl(t) : Inport  Port=4
  Atan2 : Trigonometry  Operator=atan2
  Sum : Sum  Inputs=+-
  Sum1 : Sum  Inputs=+-
  theta(t) : Outport
  wires:
  yt0(t)/1 -> Sum/1
  yl(t)/1 -> Sum/2
  xl(t)/1 -> Sum1/1
  xt(t)/1 -> Sum1/2
  Sum1/1 -> Atan2/1  "xl-xt"
  Sum/1 -> Atan2/2  "yl-yt"
  Atan2/1 -> theta(t)/1

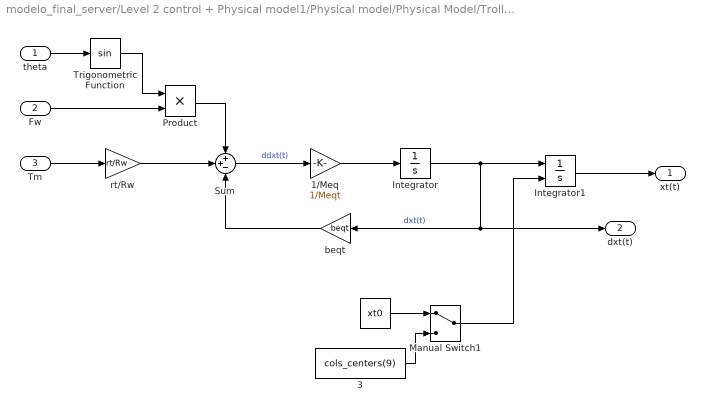
== system modelo_final_server/Level 2 control + Physical model1/Physical model/Physical Model/Trolley (carro) ==
  theta : Inport
  Fw : Inport  Port=2
  Tm : Inport  Port=3
  "   " : Constant  Value=xt0
  "   3" : Constant  Value=cols_centers(9)
  1/Meq : Gain  Gain=1/Meqt
  Integrator : Integrator
  Integrator1 : Integrator  InitialConditionSource=external
  Manual Switch1 : ManualSwitch
  Product : Product
  Sum : Sum  Inputs=++-
  Trigonometric Function : Trigonometry
  beqt : Gain  Gain=beqt
  rt/Rw : Gain  Gain=rt/Rw
  xt(t) : Outport
  dxt(t) : Outport  Port=2
  wires:
  theta/1 -> Trigonometric Function/1
  Trigonometric Function/1 -> Product/1
  Fw/1 -> Product/2
  Product/1 -> Sum/1
  Tm/1 -> rt/Rw/1
  rt/Rw/1 -> Sum/2
  Sum/1 -> 1/Meq/1  "ddxt(t)"
  1/Meq/1 -> Integrator/1
  Integrator/1 -> Integrator1/1, dxt(t)/1, beqt/1  "dxt(t)"
  beqt/1 -> Sum/3
  Integrator1/1 -> xt(t)/1
  "   "/1 -> Manual Switch1/1
  "   3"/1 -> Manual Switch1/2
  Manual Switch1/1 -> Integrator1/2

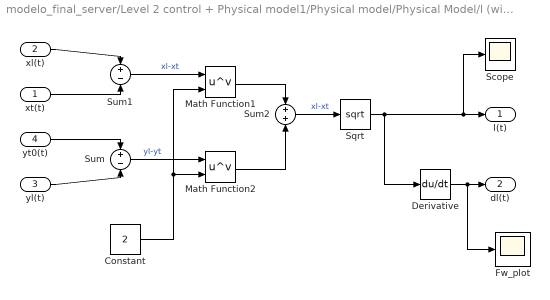
== system modelo_final_server/Level 2 control + Physical model1/Physical model/Physical Model/l (wire length) ==
  xt(t) : Inport
  xl(t) : Inport  Port=2
  yl(t) : Inport  Port=3
  yt0(t) : Inport  Port=4
  Constant : Constant  Value=2
  Derivative : Derivative
  Fw_plot : Scope
  Math Function1 : Math  Operator=pow  SignedPower=on  SaturateOnIntegerOverflow=on
  Math Function2 : Math  Operator=pow  SignedPower=on  SaturateOnIntegerOverflow=on
  Scope : Scope
  Sqrt : Sqrt  SaturateOnIntegerOverflow=on
  Sum : Sum  Inputs=+-
  Sum1 : Sum  Inputs=+-
  Sum2 : Sum
  l(t) : Outport
  dl(t) : Outport  Port=2
  wires:
  yt0(t)/1 -> Sum/1
  yl(t)/1 -> Sum/2
  xl(t)/1 -> Sum1/1
  xt(t)/1 -> Sum1/2
  Sqrt/1 -> Derivative/1, Scope/1, l(t)/1
  Sum1/1 -> Math Function1/1  "xl-xt"
  Sum/1 -> Math Function2/1  "yl-yt"
  Math Function1/1 -> Sum2/1
  Math Function2/1 -> Sum2/2
  Sum2/1 -> Sqrt/1  "xl-xt"
  Constant/1 -> Math Function2/2, Math Function1/2
  Derivative/1 -> Fw_plot/1, dl(t)/1

== matlab function modelo_final_server/MATLAB Function ==
  data: triangulo_1 output; o_2 output; x_3 output; cuadrado_4 output; u input; L1 output; R1 output; L2 output; R2 output
function [triangulo_1, o_2, x_3, cuadrado_4, L1, R1, L2, R2] = buttonMap(u)
    triangulo_1 = double(bitand(u, 1));
    
    u = bitshift(u, -1);
    o_2 = double(bitand(u, 1));
    
    u = bitshift(u, -1);
    x_3 = double(bitand(u, 1));
    
    u = bitshift(u, -1);
    cuadrado_4 = double(bitand(u, 1));
    
    u = bitshift(u, -1);
    L1 = double(bitand(u, 1));
    
    u = bitshift(u, -1);
    R1 = double(not(bitand(u, 1)));
    
    u = bitshift(u, -1);
    L2 = double(bitand(u, 1));
    
    u = bitshift(u, -1);
    R2 = double(bitand(u, 1));
end

== matlab function modelo_final_server/Level 2 control + Physical model1/Physical model/Physical Model/Mass estimation/MATLAB Function1 ==
  settings: updateMethod=DISCRETE
  data: r input; t_clock input; time output; flag_mass output; flag_int output
function [time,flag_mass, flag_int]= delay(r,t_clock)
persistent t_;
if isempty(t_) || t_clock==0
    t_ = 0;
end
persistent t_r;
if isempty(t_r) || t_clock==0
    t_r = 0;
end
persistent r_r;
if isempty(r_r) || t_clock==0
    r_r = 0;
end
if r>0.07 && r_r==0 && t_clock>=1   
   t_r=t_clock;
   r_r=1;
end
if r<=0.07
    r_r=0;
end
time_r=t_clock-t_r;
if time_r>=4.5 && t_r~=0
    flag_int=1;
else
    flag_int=0;
end
if time_r>=5 && t_r~=0
    flag_mass=1;
else
    flag_mass=0;
end
if time_r==4.5 && t_r~=0
    t_=t_clock;
end
time=t_clock-t_;

end

== matlab function modelo_final_server/Level 2 control + Physical model1/Control Level 2/Balance PD/Ganancias Control ==
  data: Mt input; Kp output; ml input; Wn input; lh input; Kd output
function [Kp,Kd] = fcn(Mt,ml,Wn,lh)
    wpos = Wn*0.89;
    g=9.81;
    Kd = -lh + ( (Mt*g)/((wpos^2)*(ml+Mt)) ) ;
    Kp = 2*wpos*0.85*(lh + Kd);
end

== matlab function modelo_final_server/MATLAB Function1 ==
  data: output output; signal input
function output = rescale(signal)

output = 0;
if signal >= 0.5 || signal < -0.5
   output = signal;
end

end

== matlab function modelo_final_server/MATLAB Function2 ==
  data: output output; signal input
function output = rescale(signal)

output = 0;
if signal >= 0.5 || signal < -0.5
   output = signal;
end

end

== matlab function modelo_final_server/Level 2 control + Physical model1/Physical model/get_obstacles_profile ==
  data: xl input; yc0xt output; cols_centers input; cols_height input; ml input; xmax input
function yc0xt = getYc0x(xl,cols_centers,cols_height, ml,xmax)
%{
@type MATLAB function called from SIMULINK
@name get_obstacles_profile
@description - Obtiene el perfil de obstaculos 
@params {float,simulation} xl - valor en tiempo real de la posocion del
carro
@params {array} cols_centers - Contiene las coordenadas de los centros de
cada columna. Array de 1xN , con N = cantidad de columnas
@params {cols_heights} - Altura de cada columna respecto del punto 0,0.
@returns {float} yc0xt - Valor en altura del obstaculo para la coordenada
xl, en el instante de tiempo t actual.
%}

yc0xt = 2.6;
aux = 0;
indice = 1;
C_WIDTH = 2.5;
%{
if(xl <= 0)
    yc0xt = 0;
    
elseif (xl >= xmax)
    yc0xt = 0;
    
elseif (xl > 0)
   for i=1:length(cols_centers)
       % xl hasta centro columna
       x_comp = xl-cols_centers(i);
        if(x_comp>= -C_WIDTH && x_comp<0)
            if (i ~= 1 && cols_height(i-1)>=cols_height(i))
                indice = i-1;
            else
                indice = i;
            end
        elseif(x_comp == 0)
            indice = i;
        elseif(x_comp<= C_WIDTH && x_comp>0)
            if (i ~= length(cols_centers) && cols_height(i+1)>=cols_height(i))
                indice = i+1;
            else
                indice = i;
            end
        end 
    end
    yc0xt=cols_height(indice);
end

if(ml > 17000) % Si el spreader esta cargado
    yc0xt = yc0xt + C_WIDTH/2;
end
%}

if(xl <= 0)
    yc0xt = 0;
    
elseif (xl >= xmax)
    yc0xt = 0;
    
elseif (xl > 0)
   for i=1:length(cols_centers)
       % xl hasta centro columna
       x_comp = abs(xl-cols_centers(i));
        if(x_comp<C_WIDTH)
           indice = i;
           break;
        elseif(x_comp == 0)
            indice = i;
            break;
        end
   end
    yc0xt=cols_height(indice);
end

end %end function

== matlab function modelo_final_server/Level 2 control + Physical model1/SWITCHES_FDC/MATLAB Function ==
  data: xt input; fdct_l output; fdct_r output
function [fdct_l,fdct_r] = fcn(xt)
fdct_l = 0;
fdct_r = 0;

if (xt > 51)
    fdct_r = 1;
elseif (xt < -28)
        fdct_l = 1;
end
end

== matlab function modelo_final_server/Level 2 control + Physical model1/SWITCHES_FDC/MATLAB Function1 ==
  data: lh input; fdch_up output; fdch_down output
function [fdch_up,fdch_down] = fcn(lh)
fdch_up = 0;
fdch_down = 0;

if (lh > 51)
    fdch_down = 1;
elseif (lh <= 0)
        fdch_up = 1;
end

end
